simulink model "vis_servo_TR"  (R2020b)
settings: Solver=ode45  StartTime=0.0  StopTime=1000  MaxStep=.5e-3  RelTol=1e-8
InitFcn:
  | init
values from neighbouring files (symbols this model uses):
  s_star_end = C_features_desired(:)    [init.m]
  W_T_C_0 = W_T_C_desired*SE3(R_0, t_0)    [init.m]
  W_T_C_desired = W_T_O*O_T_C_desired    [init.m]
undefined symbols (not defined in the file or in its folder): rotm2quat, s_eq3
settings Model: Creator=marco  LastModifiedBy=marco

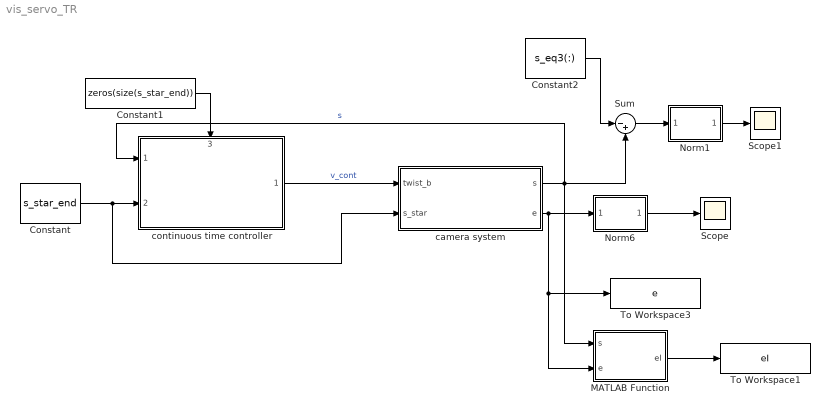
== system vis_servo_TR ==
  Constant : Constant  Value=s_star_end
  Constant1 : Constant  Value=zeros(size(s_star_end))
  Constant2 : Constant  Value=s_eq3(:)
  MATLAB Function : MATLAB Function  TreatAsAtomicUnit=on
  Norm1 : Subsystem  ReferencedSubsystem=Norm
  Norm6 : Subsystem  ReferencedSubsystem=Norm
  Scope : Scope
  Scope1 : Scope
  Sum : Sum  Inputs=|-+
  To Workspace1 : ToWorkspace  VariableName=eI  SaveFormat=Timeseries  SampleTime=0.001
  To Workspace3 : ToWorkspace  VariableName=e  SaveFormat=Timeseries  SampleTime=0.001
  camera system : Subsystem  mask{W_p_C_0=W_T_C_0.t, W_q_C_0=rotm2quat(W_T_C_0.R)', s_star_end=s_star_end, W_T_Cd=W_T_C_desired.double}
  continuous time controller : Subsystem  ReferencedSubsystem=continuous_time_controller  lambda=10  forward_action_enabled=off
      settings: PortSchema="{\"entries\":[{\"content\":{\"sides\":[{\"content\":{\"connectorIds\":[\"In1\",\"In2\"]},\"type\":\"ConnectorPlacement.EquallySpacedRectSide\",\"uuid\":\"e89226d4-baa4-4c30-af13-ff098f2ce7fc\"},{\"content\":{\"connectorIds\":[\"Out1\"],\"side\":\"RIGHT\"},\"type\":\"ConnectorPlacement.EquallySpacedRectSide\",\"uuid\":\"9d8bce32-3e74-4b83-8e79-37f4d5184f5a\"},{\"content\":{\"connectorIds\":[\"In3\"],\"side\":\"TOP\"},\"type\":\"ConnectorPlacement.EquallySpacedRectSide\",\"uuid\":\"9322580e-0316-476d-a1f3-db89d995a642\"},{\"content\":{\"connectorIds\":[],\"side\":\"HIDDEN\"},\"type\":\"ConnectorPlacement.EquallySpacedRectSide\",\"uuid\":\"a71e587c-d25e-434f-ae20-c6224730a5c7\"}]},\"type\":\"ConnectorPlacement.EquallySpacedConnector\",\"uuid\":\"c231d1ba-4204-4ba1-a9fd-ba17f6d657c2\"}],\"packageUris\":[\"http://schema.mathworks.com/mf0/Connector/R2020b\"],\"version\":\"1.0\"}"
  wires:
  Constant/1 -> camera system/2(s_star), continuous time controller/2
  camera system/1(s) -> Sum/2, MATLAB Function/1(s), continuous time controller/1  "s"
  continuous time controller/1 -> camera system/1(twist_b)  "v_cont"
  Constant1/1 -> continuous time controller/3
  camera system/2(e) -> MATLAB Function/2(e), To Workspace3/1, Norm6/1
  Norm6/1 -> Scope/1
  MATLAB Function/1(eI) -> To Workspace1/1
  Constant2/1 -> Sum/1
  Sum/1 -> Norm1/1
  Norm1/1 -> Scope1/1

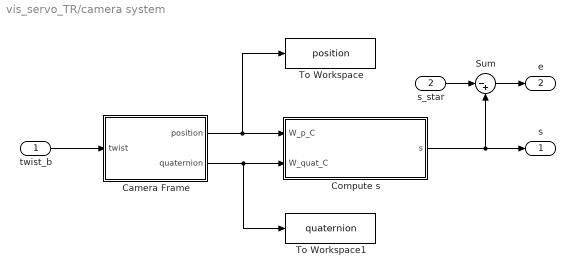
== system vis_servo_TR/camera system ==
  twist_b : Inport
  s_star : Inport  Port=2
  Camera Frame : Subsystem
  Compute s : MATLAB Function  TreatAsAtomicUnit=on
  Sum : Sum  Inputs=|-+
  To Workspace : ToWorkspace  VariableName=position  SaveFormat=Timeseries  SampleTime=0.001
  To Workspace1 : ToWorkspace  VariableName=quaternion  SaveFormat=Timeseries  SampleTime=0.001
  s : Outport
  e : Outport  Port=2
  wires:
  Camera Frame/1(position) -> To Workspace/1, Compute s/1(W_p_C)
  Camera Frame/2(quaternion) -> To Workspace1/1, Compute s/2(W_quat_C)
  twist_b/1 -> Camera Frame/1(twist)
  Compute s/1(s) -> Sum/2, s/1
  Sum/1 -> e/1
  s_star/1 -> Sum/1

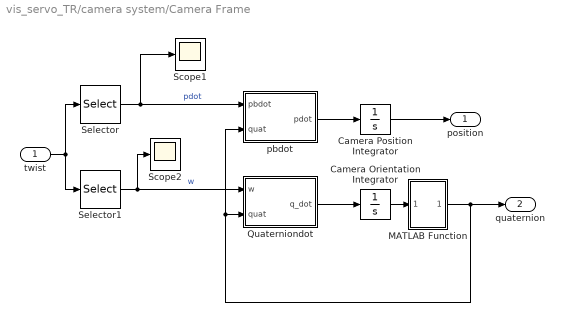
== system vis_servo_TR/camera system/Camera Frame ==
  twist : Inport
  Camera Orientation Integrator : Integrator  InitialCondition=W_q_C_0
  Camera Position Integrator : Integrator  InitialCondition=W_p_C_0
  MATLAB Function : MATLAB Function  TreatAsAtomicUnit=on
  Quaterniondot : MATLAB Function  TreatAsAtomicUnit=on
  Scope1 : Scope
  Scope2 : Scope
  Selector : Selector  InputPortWidth=6  IndexOptions=Index vector (dialog)  Indices=[1:3]  OutputSizes=1
  Selector1 : Selector  InputPortWidth=6  IndexOptions=Index vector (dialog)  Indices=[4:6]  OutputSizes=1
  pbdot : MATLAB Function  TreatAsAtomicUnit=on
  position : Outport
  quaternion : Outport  Port=2
  wires:
  twist/1 -> Selector/1, Selector1/1
  Selector/1 -> Scope1/1, pbdot/1(pbdot)  "pdot"
  Selector1/1 -> Scope2/1, Quaterniondot/1(w)  "w"
  Camera Position Integrator/1 -> position/1
  Quaterniondot/1(q_dot) -> Camera Orientation Integrator/1
  Camera Orientation Integrator/1 -> MATLAB Function/1("quat ")
  pbdot/1(pdot) -> Camera Position Integrator/1
  MATLAB Function/1(quat) -> quaternion/1, pbdot/2(quat), Quaterniondot/2(quat)

== matlab function vis_servo_TR/MATLAB Function ==
  data: s input; eI output; e input
function eI = fcn(s, e)

L = computeL(s);
eI = L*pinv(L)*e;

== matlab function vis_servo_TR/camera system/Camera Frame/MATLAB Function ==
  data: quat input; quat output
function quat = fcn(quat)

quat = unit(quat);

== matlab function vis_servo_TR/camera system/Camera Frame/Quaterniondot ==
  data: w input; q_dot output; quat input
function q_dot = fcn(w, quat)

q_dot = quat_dotb(quat,w);
% Q = UnitQuaternion(quat);
% Q_dot = Q.dot(w);
% q_dot = Q_dot.double'; 
% q_dot = [0 0 0 0]';

== matlab function vis_servo_TR/camera system/Camera Frame/pbdot ==
  data: pbdot input; pdot output; quat input
function pdot = fcn(pbdot, quat)

W_R_B = quat2rotm(quat');
pdot = W_R_B*pbdot;

== matlab function vis_servo_TR/camera system/Compute s ==
  data: W_p_C input; s output; W_quat_C input; s_star_end parameter; W_T_Cd parameter
function s = fcn(W_p_C, W_quat_C, s_star_end, W_T_Cd)

% W_T_C = SE3(quat2rotm(W_quat_C'),W_p_C);
W_T_C = [quat2rotm(W_quat_C'), W_p_C; 0 0 0 1];

% C_features = inv(W_T_C) * params.W_T_O * params.O_features;
C_T_Cd = invSE3(W_T_C) * W_T_Cd;
C_features = zeros(3,numel(s_star_end)/3);
C_features = homtrans(C_T_Cd, reshape(s_star_end,3,numel(s_star_end)/3));

s = C_features(:);

% s = params.O_features(:);
